simulink model "penerima_bpsk"  (R2022a)
settings: Solver=FixedStepDiscrete  StartTime=0.0  StopTime=10.0  RelTol=1e-3
libraries: commchan3 x1, embmathops x1, commrandsrc3 x1
settings Model: DataTypeOverride=Off  Creator=acer  LastModifiedBy=acer
settings OptimizationCC: BlockReduction=off  ConditionallyExecuteInputs=off  DefaultParameterBehavior=Inlined  InheritOutputTypeSmallerThanSingle=on
settings DebuggingCC: AlgebraicLoopMsg=error  SingleTaskRateTransMsg=error
settings HardwareCC: ProdBitPerPointer=32  ProdBitPerSizeT=32  ProdBitPerPtrDiffT=32  ProdLargestAtomicFloat=None  ProdIntDivRoundTo=Undefined  ProdEndianess=Unspecified  ProdWordSize=32  ProdHWDeviceType=ASIC/FPGA->ASIC/FPGA  TargetBitPerPointer=64  TargetBitPerSizeT=64  TargetBitPerPtrDiffT=64  TargetLongLongMode=on  TargetIntDivRoundTo=Zero  TargetEndianess=LittleEndian  TargetWordSize=64  TargetHWDeviceType=Custom Processor->MATLAB Host Computer  ProdEqTarget=off

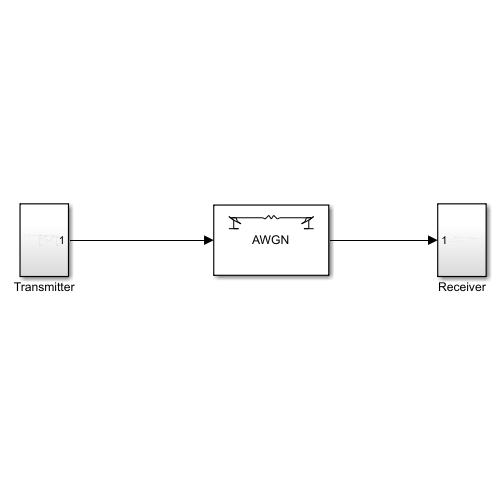
[thumbnail: Simulink's stored preview of the top-level diagram]
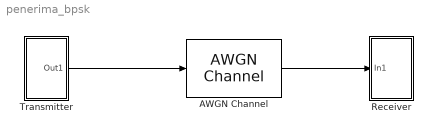
== system penerima_bpsk ==
  AWGN Channel : commchan3/AWGN Channel  InputProcessing=Columns as channels (frame based)  seed=67  noiseMode="Signal to noise ratio  (SNR)"  EbNodB=10  EsNodB=10  SNRdB=1  bitsPerSym=1  Ps=1  Tsym=1  variance=1
  Receiver : Subsystem
  Transmitter : Subsystem
  wires:
  Transmitter/1(Out1) -> AWGN Channel/1
  AWGN Channel/1 -> Receiver/1(In1)

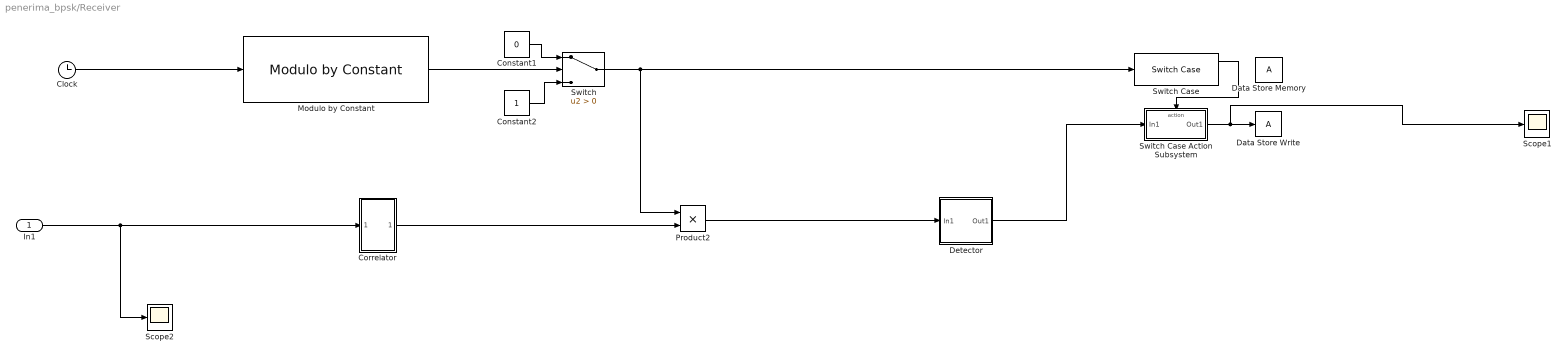
== system penerima_bpsk/Receiver ==
  In1 : Inport
  Clock : Clock
  Constant1 : Constant  Value=0
  Constant2 : Constant
  Correlator : Subsystem
  Data Store Memory : DataStoreMemory  WriteAfterWriteMsg=warning  ShowAdditionalParam=off
  Data Store Write : DataStoreWrite  IndexOptions=Index vector (dialog)  Indices=1  OutputSizes=1
  Detector : Subsystem
  Modulo by Constant : embmathops/Modulo by Constant  Denominator=1  SimulateUsing=Code generation
      settings: SourceProductBaseCode=SL
  Product2 : Product
  Scope1 : Scope
  Scope2 : Scope
  Switch : Switch  Criteria=u2 > Threshold  SaturateOnIntegerOverflow=off  InputSameDT=off
  Switch Case : SwitchCase
  Switch Case Action Subsystem : Subsystem  TreatAsAtomicUnit=on
  wires:
  In1/1 -> Scope2/1, Correlator/1(In1)
  Clock/1 -> Modulo by Constant/1
  Modulo by Constant/1 -> Switch/2
  Switch/1 -> Switch Case/1, Product2/1
  Constant2/1 -> Switch/3
  Constant1/1 -> Switch/1
  Switch Case/1 -> Switch Case Action Subsystem/Action
  Switch Case Action Subsystem/1(Out1) -> Scope1/1, Data Store Write/1
  Product2/1 -> Detector/1(In1)
  Detector/1(Out1) -> Switch Case Action Subsystem/1(In1)
  Correlator/1(Out1) -> Product2/2

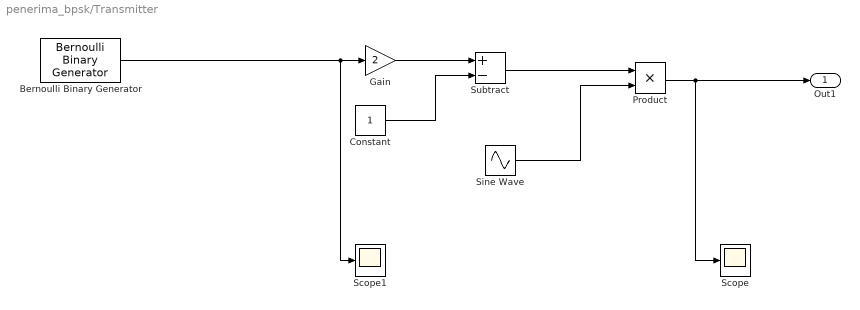
== system penerima_bpsk/Transmitter ==
  Bernoulli Binary Generator : commrandsrc3/Bernoulli Binary Generator  ProbabilityOfZero=0.5  SeedSource=Parameter  Seed=32  SampleTime=1  SamplesPerFrame=1  OutputDataType=double  SimulateUsing=Interpreted execution
  Constant : Constant
  Gain : Gain  Gain=2
  Product : Product
  Scope : Scope
  Scope1 : Scope
  Sine Wave : Sin  Amplitude=sqrt(2)  Frequency=2*pi  Phase=0.5*pi  SampleTime=0.01
  Subtract : Sum  Inputs=+-
  Out1 : Outport
  wires:
  Product/1 -> Out1/1, Scope/1
  Sine Wave/1 -> Product/2
  Bernoulli Binary Generator/1 -> Scope1/1, Gain/1
  Subtract/1 -> Product/1
  Constant/1 -> Subtract/2
  Gain/1 -> Subtract/1

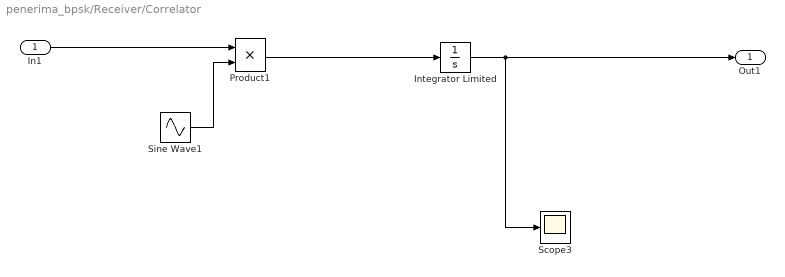
== system penerima_bpsk/Receiver/Correlator ==
  In1 : Inport
  Integrator Limited : Integrator  LimitOutput=on  UpperSaturationLimit=1  LowerSaturationLimit=0
  Product1 : Product
  Scope3 : Scope
  Sine Wave1 : Sin  Amplitude=sqrt(2)  Frequency=2*pi  Phase=0.5*pi  SampleTime=0.01
  Out1 : Outport
  wires:
  In1/1 -> Product1/1
  Integrator Limited/1 -> Out1/1, Scope3/1
  Sine Wave1/1 -> Product1/2
  Product1/1 -> Integrator Limited/1

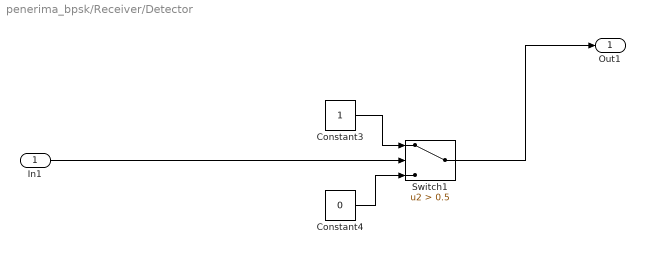
== system penerima_bpsk/Receiver/Detector ==
  In1 : Inport
  Constant3 : Constant
  Constant4 : Constant  Value=0
  Switch1 : Switch  Criteria=u2 > Threshold  Threshold=0.5  SaturateOnIntegerOverflow=off  InputSameDT=off
  Out1 : Outport
  wires:
  In1/1 -> Switch1/2
  Constant4/1 -> Switch1/3
  Switch1/1 -> Out1/1
  Constant3/1 -> Switch1/1

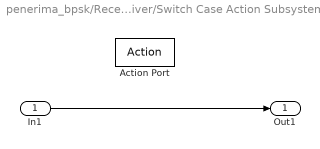
== system penerima_bpsk/Receiver/Switch Case Action Subsystem ==
  In1 : Inport
  Action Port : ActionPort  ActionPortLabel=case [ 1 ]:
  Out1 : Outport
  wires:
  In1/1 -> Out1/1
